simulink model "multirotor_simulation"  (R2025b)
settings: Solver=ode4  StartTime=0.0  StopTime=21  FixedStep=ST  RelTol=1e-3
values from neighbouring files (symbols this model uses):
  a0 = 0    [multirotor_start.m]
  ASLOPE = 5.9    [multirotor_start.m]
  Ax = 0.023    [multirotor_start.m]
  Ay = 0.023    [multirotor_start.m]
  Az = 0.106    [multirotor_start.m]
  BLADES = 2    [multirotor_start.m]
  BLCG = 0    [multirotor_start.m]
  BLCP = 0    [multirotor_start.m]
  BLH1 = b*sind(30)    [multirotor_start.m]
  BLH2 = b    (= 0.275)    [multirotor_start.m]
  BLH3 = b*sind(30)    [multirotor_start.m]
  BLH4 = -b*sind(30)    [multirotor_start.m]
  BLH5 = -b    (= -0.275)    [multirotor_start.m]
  BLH6 = -b*sind(30)    [multirotor_start.m]
  chi1 = 1    [multirotor_start.m]
  chi2 = -1    [multirotor_start.m]
  chi3 = 1    [multirotor_start.m]
  chi4 = -1    [multirotor_start.m]
  chi5 = 1    [multirotor_start.m]
  chi6 = -1    [multirotor_start.m]
  CHORD = 17.55e-3    (= 0.01755)    [multirotor_start.m]
  CHORD75 = 21e-3    (= 0.021)    [multirotor_start.m]
  controller_mode = 1    [multirotor_start.m]
  del_sp = [0 0.7 0 0]'    [multirotor_start.m]
  dyn_visco = 17.89e-6    (= 1.789e-05)    [multirotor_start.m]
  g0 = 9.80665    [multirotor_start.m]
  href = 0    [multirotor_start.m]
  k_ind = 1.35    [multirotor_start.m]
  k_Omega = 14.92    [multirotor_start.m]
  latref = 44.200626    [multirotor_start.m]
  lonref = 12.063822    [multirotor_start.m]
  m = 2.15    [multirotor_start.m]
  MC_ATT_PITCH = 30*pi/180    (= 0.523598775598)    [multirotor_start.m]
  MC_ATT_ROLL = 30*pi/180    (= 0.523598775598)    [multirotor_start.m]
  MC_ATT_YAW = 180*pi/180    (= 3.14159265359)    [multirotor_start.m]
  MC_PITCH_P = 3    [multirotor_start.m]
  MC_PITCHRATE_D = 0    [multirotor_start.m]
  MC_PITCHRATE_I = 0.1*0.5    (= 0.05)    [multirotor_start.m]
  MC_PITCHRATE_P = 0.09    [multirotor_start.m]
  MC_ROLL_P = 3    [multirotor_start.m]
  MC_ROLLRATE_D = 0    [multirotor_start.m]
  MC_ROLLRATE_I = 0.1*0.5    (= 0.05)    [multirotor_start.m]
  MC_ROLLRATE_P = 0.09    [multirotor_start.m]
  MC_VEL_FWD = 5    [multirotor_start.m]
  MC_VEL_FWD_OPT = 0.5    [multirotor_start.m]
  MC_VEL_LAT = 5    [multirotor_start.m]
  MC_VEL_LAT_OPT = 0.5    [multirotor_start.m]
  MC_VEL_VERT = 1    [multirotor_start.m]
  MC_YAW_P = 1.8*0.5    (= 0.9)    [multirotor_start.m]
  MC_YAWRATE_D = 0    [multirotor_start.m]
  MC_YAWRATE_I = 0.1*0    (= 0)    [multirotor_start.m]
  MC_YAWRATE_P = 0.175*0.4    (= 0.07)    [multirotor_start.m]
  MPC_XY_VEL_D_ACC = 0.2*2    (= 0.4)    [multirotor_start.m]
  MPC_XY_VEL_I_ACC = 0.8    [multirotor_start.m]
  MPC_XY_VEL_P_ACC = 1.7*3/3    (= 1.7)    [multirotor_start.m]
  MPC_Z_VEL_D_ACC = 0    [multirotor_start.m]
  MPC_Z_VEL_I_ACC = 2    [multirotor_start.m]
  MPC_Z_VEL_P_ACC = 4    [multirotor_start.m]
  n = 0.6359    [multirotor_start.m]
  p00 = 7.145e-2    (= 0.07145)    [multirotor_start.m]
  p01 = 0.4377    [multirotor_start.m]
  p02 = -10.13    [multirotor_start.m]
  p10 = 1.259e-3    (= 0.001259)    [multirotor_start.m]
  p11 = 1.284e-3    (= 0.001284)    [multirotor_start.m]
  p20 = -7.513e-7    (= -7.513e-07)    [multirotor_start.m]
  PWM_hover = (PWM_idle+PWM_max)/2    (= 1550)    [multirotor_start.m]
  PWM_idle = 1100    [multirotor_start.m]
  PWM_max = 2000    [multirotor_start.m]
  ROTOR = 4*0.0254    (= 0.1016)    [multirotor_start.m]
  set_point_input = 0    [multirotor_start.m]
  ST = 0.01    [multirotor_start.m]
  STACG = 0    [multirotor_start.m]
  STACP = 0    [multirotor_start.m]
  STAH1 = -b*cosd(30)    [multirotor_start.m]
  STAH2 = 0    [multirotor_start.m]
  STAH3 = b*cosd(30)    [multirotor_start.m]
  STAH4 = b*cosd(30)    [multirotor_start.m]
  STAH5 = 0    [multirotor_start.m]
  STAH6 = -b*cosd(30)    [multirotor_start.m]
  TERMINAL_SPEED = 0.5    [multirotor_start.m]
  Theta0 = 45*pi/180    (= 0.785398163397)    [multirotor_start.m]
  THETT = -38.0973*pi/180    (= -0.66492332112)    [multirotor_start.m]
  V_sin_x = 0.3    [multirotor_start.m]
  Vsp = [0 1 0]'    [multirotor_start.m]
  wind_rate = [0 0 0]'    [multirotor_start.m]
  wind_velocity_e = [0 0 0]'    [multirotor_start.m]
  WLCG = -0.03    [multirotor_start.m]
  WLCP = -0.08    [multirotor_start.m]
  WLH1 = 32e-3    (= 0.032)    [multirotor_start.m]
  WLH2 = 32e-3    (= 0.032)    [multirotor_start.m]
  WLH3 = 32e-3    (= 0.032)    [multirotor_start.m]
  WLH4 = 32e-3    (= 0.032)    [multirotor_start.m]
  WLH5 = 32e-3    (= 0.032)    [multirotor_start.m]
  WLH6 = 32e-3    (= 0.032)    [multirotor_start.m]
  Xe_target = Xe_0 + [2, 3, -10]'    [multirotor_start.m]
undefined symbols (not defined in the file or in its folder): fspecial, gray, Rec, SDTV, Sim3dSensor, X, Y, Z
libraries: sm_lib x258, slpidlib x18, nesl_utility x15, sharedtransform x4, simulink x3, aerolibanimutils x2, sim3dcameralib x2, dspvision x2, uavsim3dlib x2, aerolibutil x2, visionconversions x1, visionanalysis x1
(part 9 of 10)

== system multirotor_simulation/MULTIROTOR/3D/SIMECHANICS 3D SCENE/SimMechanics/MotorC/DCBL_Assembly_Clockwise_3_Top_1_RIGID/Assem3DCBL_Assembly_Clockwise_3_Top_1_RIGID ==
  Mieng_chan_canh_quat_1_RIGID : Subsystem
  ReferenceFrame : sm_lib/Frames and Transforms/Reference Frame
  Tang_tren_DCBL_1_RIGID : Subsystem
  Transform : sm_lib/Frames and Transforms/Rigid Transform  TranslationMethod=None  TranslationStandardOffset=0  TranslationStandardOffsetUnits=m  TranslationStandardAxis=+Z  TranslationCartesianOffset=[0 0 0]  TranslationCartesianOffsetUnits=m  TranslationROffset=0  TranslationROffsetUnits=m  TranslationZOffset=0  TranslationZOffsetUnits=m  TranslationThetaOffset=0  TranslationThetaOffsetUnits=deg  RotationMethod=None  RotationAngleUnits=deg  RotationStandardAxis=+Z  RotationAngle=0  RotationArbitraryAxis=[0 0 1]  FollAlignAxisA=+X  BaseAlignAxisA=+Y  FollAlignAxisB=+Y  BaseAlignAxisB=+Z  RotationSequenceAxes=FollowerAxes  RotationSequence=XYX  RotationSequenceAngles=[0 0 0]  RotationSequenceAnglesUnits=deg  RotationMatrix=[1 0 0; 0 1 0; 0 0 1]  Quaternion=[1 0 0 0]
  Transform1 : sm_lib/Frames and Transforms/Rigid Transform  TranslationMethod=Cartesian  TranslationStandardOffset=0  TranslationStandardOffsetUnits=mm  TranslationStandardAxis=+Z  TranslationCartesianOffset=[5.0000000000000044 5.5000000000000053 3.8000000000000256]  TranslationCartesianOffsetUnits=mm  TranslationROffset=0  TranslationROffsetUnits=m  TranslationZOffset=0  TranslationZOffsetUnits=m  TranslationThetaOffset=0  TranslationThetaOffsetUnits=deg  RotationMethod=ArbitraryAxis  RotationAngleUnits=rad  RotationStandardAxis=+Z  RotationAngle=3.1415926535897931  RotationArbitraryAxis=[0 1 0]  FollAlignAxisA=+X  BaseAlignAxisA=+Y  FollAlignAxisB=+Y  BaseAlignAxisB=+Z  RotationSequenceAxes=FollowerAxes  RotationSequence=XYX  RotationSequenceAngles=[0 0 0]  RotationSequenceAnglesUnits=deg  RotationMatrix=[1 0 0; 0 1 0; 0 0 1]  Quaternion=[1 0 0 0]
  Transform2 : sm_lib/Frames and Transforms/Rigid Transform  TranslationMethod=Cartesian  TranslationStandardOffset=0  TranslationStandardOffsetUnits=mm  TranslationStandardAxis=+Z  TranslationCartesianOffset=[0 12.200000000000017 0]  TranslationCartesianOffsetUnits=mm  TranslationROffset=0  TranslationROffsetUnits=m  TranslationZOffset=0  TranslationZOffsetUnits=m  TranslationThetaOffset=0  TranslationThetaOffsetUnits=deg  RotationMethod=ArbitraryAxis  RotationAngleUnits=rad  RotationStandardAxis=+Z  RotationAngle=3.1415926535897931  RotationArbitraryAxis=[0 1 0]  FollAlignAxisA=+X  BaseAlignAxisA=+Y  FollAlignAxisB=+Y  BaseAlignAxisB=+Z  RotationSequenceAxes=FollowerAxes  RotationSequence=XYX  RotationSequenceAngles=[0 0 0]  RotationSequenceAnglesUnits=deg  RotationMatrix=[1 0 0; 0 1 0; 0 0 1]  Quaternion=[1 0 0 0]
  Transform3 : sm_lib/Frames and Transforms/Rigid Transform  TranslationMethod=Cartesian  TranslationStandardOffset=0  TranslationStandardOffsetUnits=mm  TranslationStandardAxis=+Z  TranslationCartesianOffset=[0 16.899999999999999 0]  TranslationCartesianOffsetUnits=mm  TranslationROffset=0  TranslationROffsetUnits=m  TranslationZOffset=0  TranslationZOffsetUnits=m  TranslationThetaOffset=0  TranslationThetaOffsetUnits=deg  RotationMethod=ArbitraryAxis  RotationAngleUnits=rad  RotationStandardAxis=+Z  RotationAngle=2.0943951023931957  RotationArbitraryAxis=[-0.57735026918962562 0.57735026918962573 0.57735026918962573]  FollAlignAxisA=+X  BaseAlignAxisA=+Y  FollAlignAxisB=+Y  BaseAlignAxisB=+Z  RotationSequenceAxes=FollowerAxes  RotationSequence=XYX  RotationSequenceAngles=[0 0 0]  RotationSequenceAnglesUnits=deg  RotationMatrix=[1 0 0; 0 1 0; 0 0 1]  Quaternion=[1 0 0 0]
  Transform4 : sm_lib/Frames and Transforms/Rigid Transform  TranslationMethod=Cartesian  TranslationStandardOffset=0  TranslationStandardOffsetUnits=mm  TranslationStandardAxis=+Z  TranslationCartesianOffset=[0 30.500000000000014 0]  TranslationCartesianOffsetUnits=mm  TranslationROffset=0  TranslationROffsetUnits=m  TranslationZOffset=0  TranslationZOffsetUnits=m  TranslationThetaOffset=0  TranslationThetaOffsetUnits=deg  RotationMethod=ArbitraryAxis  RotationAngleUnits=rad  RotationStandardAxis=+Z  RotationAngle=2.994911156014171  RotationArbitraryAxis=[0 1 0]  FollAlignAxisA=+X  BaseAlignAxisA=+Y  FollAlignAxisB=+Y  BaseAlignAxisB=+Z  RotationSequenceAxes=FollowerAxes  RotationSequence=XYX  RotationSequenceAngles=[0 0 0]  RotationSequenceAnglesUnits=deg  RotationMatrix=[1 0 0; 0 1 0; 0 0 1]  Quaternion=[1 0 0 0]
  hex_nut_style_1_gradeab_iso_1_RIGID : Subsystem
  x10x4_7_clockwise_propeller_1_RIGID : Subsystem
  F : PMIOPort  Side=Left
  connections:
  Tang_tren_DCBL_1_RIGID/LConn1 -- Transform/RConn1
  Transform1/RConn1 -- x10x4_7_clockwise_propeller_1_RIGID/LConn1
  Mieng_chan_canh_quat_1_RIGID/LConn1 -- Transform2/RConn1
  Transform3/RConn1 -- hex_nut_style_1_gradeab_iso_1_RIGID/LConn1
  Transform/LConn1 -- ReferenceFrame/RConn1 -- Transform1/LConn1 -- Transform2/LConn1 -- Transform3/LConn1 -- Transform4/RConn1
  Transform4/LConn1 -- F/RConn1

== system multirotor_simulation/MULTIROTOR/3D/SIMECHANICS 3D SCENE/SimMechanics/MotorD/DCBL_Assembly_CounterClockwise_4_Top_1_RIGID/Assem4DCBL_Assembly_CounterClockwise_4_Top_1_RIGID ==
  Mieng_chan_canh_quat_1_RIGID : Subsystem
  ReferenceFrame : sm_lib/Frames and Transforms/Reference Frame
  Tang_tren_DCBL_1_RIGID : Subsystem
  Transform : sm_lib/Frames and Transforms/Rigid Transform  TranslationMethod=None  TranslationStandardOffset=0  TranslationStandardOffsetUnits=m  TranslationStandardAxis=+Z  TranslationCartesianOffset=[0 0 0]  TranslationCartesianOffsetUnits=m  TranslationROffset=0  TranslationROffsetUnits=m  TranslationZOffset=0  TranslationZOffsetUnits=m  TranslationThetaOffset=0  TranslationThetaOffsetUnits=deg  RotationMethod=None  RotationAngleUnits=deg  RotationStandardAxis=+Z  RotationAngle=0  RotationArbitraryAxis=[0 0 1]  FollAlignAxisA=+X  BaseAlignAxisA=+Y  FollAlignAxisB=+Y  BaseAlignAxisB=+Z  RotationSequenceAxes=FollowerAxes  RotationSequence=XYX  RotationSequenceAngles=[0 0 0]  RotationSequenceAnglesUnits=deg  RotationMatrix=[1 0 0; 0 1 0; 0 0 1]  Quaternion=[1 0 0 0]
  Transform1 : sm_lib/Frames and Transforms/Rigid Transform  TranslationMethod=Cartesian  TranslationStandardOffset=0  TranslationStandardOffsetUnits=mm  TranslationStandardAxis=+Z  TranslationCartesianOffset=[0 12.200000000000017 0]  TranslationCartesianOffsetUnits=mm  TranslationROffset=0  TranslationROffsetUnits=m  TranslationZOffset=0  TranslationZOffsetUnits=m  TranslationThetaOffset=0  TranslationThetaOffsetUnits=deg  RotationMethod=ArbitraryAxis  RotationAngleUnits=rad  RotationStandardAxis=+Z  RotationAngle=3.1415926535897931  RotationArbitraryAxis=[0 1 0]  FollAlignAxisA=+X  BaseAlignAxisA=+Y  FollAlignAxisB=+Y  BaseAlignAxisB=+Z  RotationSequenceAxes=FollowerAxes  RotationSequence=XYX  RotationSequenceAngles=[0 0 0]  RotationSequenceAnglesUnits=deg  RotationMatrix=[1 0 0; 0 1 0; 0 0 1]  Quaternion=[1 0 0 0]
  Transform2 : sm_lib/Frames and Transforms/Rigid Transform  TranslationMethod=Cartesian  TranslationStandardOffset=0  TranslationStandardOffsetUnits=mm  TranslationStandardAxis=+Z  TranslationCartesianOffset=[5.0000000000000044 5.5000000000000053 3.8000000000000118]  TranslationCartesianOffsetUnits=mm  TranslationROffset=0  TranslationROffsetUnits=m  TranslationZOffset=0  TranslationZOffsetUnits=m  TranslationThetaOffset=0  TranslationThetaOffsetUnits=deg  RotationMethod=ArbitraryAxis  RotationAngleUnits=rad  RotationStandardAxis=+Z  RotationAngle=3.1415926535897931  RotationArbitraryAxis=[0 1 0]  FollAlignAxisA=+X  BaseAlignAxisA=+Y  FollAlignAxisB=+Y  BaseAlignAxisB=+Z  RotationSequenceAxes=FollowerAxes  RotationSequence=XYX  RotationSequenceAngles=[0 0 0]  RotationSequenceAnglesUnits=deg  RotationMatrix=[1 0 0; 0 1 0; 0 0 1]  Quaternion=[1 0 0 0]
  Transform3 : sm_lib/Frames and Transforms/Rigid Transform  TranslationMethod=Cartesian  TranslationStandardOffset=0  TranslationStandardOffsetUnits=mm  TranslationStandardAxis=+Z  TranslationCartesianOffset=[0 16.899999999999999 0]  TranslationCartesianOffsetUnits=mm  TranslationROffset=0  TranslationROffsetUnits=m  TranslationZOffset=0  TranslationZOffsetUnits=m  TranslationThetaOffset=0  TranslationThetaOffsetUnits=deg  RotationMethod=ArbitraryAxis  RotationAngleUnits=rad  RotationStandardAxis=+Z  RotationAngle=2.0943951023931953  RotationArbitraryAxis=[-0.57735026918962584 0.57735026918962584 0.57735026918962584]  FollAlignAxisA=+X  BaseAlignAxisA=+Y  FollAlignAxisB=+Y  BaseAlignAxisB=+Z  RotationSequenceAxes=FollowerAxes  RotationSequence=XYX  RotationSequenceAngles=[0 0 0]  RotationSequenceAnglesUnits=deg  RotationMatrix=[1 0 0; 0 1 0; 0 0 1]  Quaternion=[1 0 0 0]
  Transform4 : sm_lib/Frames and Transforms/Rigid Transform  TranslationMethod=Cartesian  TranslationStandardOffset=0  TranslationStandardOffsetUnits=mm  TranslationStandardAxis=+Z  TranslationCartesianOffset=[0 30.500000000000014 0]  TranslationCartesianOffsetUnits=mm  TranslationROffset=0  TranslationROffsetUnits=m  TranslationZOffset=0  TranslationZOffsetUnits=m  TranslationThetaOffset=0  TranslationThetaOffsetUnits=deg  RotationMethod=ArbitraryAxis  RotationAngleUnits=rad  RotationStandardAxis=+Z  RotationAngle=2.994911156014171  RotationArbitraryAxis=[0 1 0]  FollAlignAxisA=+X  BaseAlignAxisA=+Y  FollAlignAxisB=+Y  BaseAlignAxisB=+Z  RotationSequenceAxes=FollowerAxes  RotationSequence=XYX  RotationSequenceAngles=[0 0 0]  RotationSequenceAnglesUnits=deg  RotationMatrix=[1 0 0; 0 1 0; 0 0 1]  Quaternion=[1 0 0 0]
  hex_nut_style_1_gradeab_iso_1_RIGID : Subsystem
  x10x4_7_counterclockwise_propeller_1_RIGID : Subsystem
  F : PMIOPort  Side=Left
  connections:
  Tang_tren_DCBL_1_RIGID/LConn1 -- Transform/RConn1
  Mieng_chan_canh_quat_1_RIGID/LConn1 -- Transform1/RConn1
  Transform2/RConn1 -- x10x4_7_counterclockwise_propeller_1_RIGID/LConn1
  Transform3/RConn1 -- hex_nut_style_1_gradeab_iso_1_RIGID/LConn1
  Transform/LConn1 -- Transform1/LConn1 -- Transform4/RConn1 -- ReferenceFrame/RConn1 -- Transform2/LConn1 -- Transform3/LConn1
  Transform4/LConn1 -- F/RConn1

== system multirotor_simulation/MULTIROTOR/3D/SIMECHANICS 3D SCENE/SimMechanics/Assembly_Quadrotor_NProp_1_RIGID/Assembly_Quadrotor_NoProp_1_RIGID/DCBL_Assembly_Clockwise_1_Bottom_1_RIGID/De_DCBL_1_RIGID ==
  ReferenceFrame : sm_lib/Frames and Transforms/Reference Frame
  Solid : sm_lib/Body Elements/File Solid  ExtGeomFileName=De_DCBL_Default_sldprt.STL  UnitType=Custom  ExtGeomFileUnits=mm  StepReaderType=HEX  ExportConvexHullGeometry=off  InertiaType=Custom  Mass=0.0094405067370886605  MassUnits=kg  CenterOfMass=[0 8.551755407943574 0]  CenterOfMassUnits=mm  MomentsOfInertia=[0.9581719720589793 0.57744869492610285 0.95817197205897908]  MomentsOfInertiaUnits=kg*mm^2  ProductsOfInertia=[0 -0.0012524646336928653 0]  ProductsOfInertiaUnits=kg*mm^2  BasedOnType=Density  Density=1000  DensityUnits=kg/(m^3)  DoExposeReferenceFrame=on  SerializedFrames=<Frames/>  GraphicType=FromGeometry  MarkerShape=Sphere  MarkerSize=10  MarkerSizeUnits=m  GraphicVisPropType=SimpleVisualProperties  GraphicDiffuseColor=[0.2 0.2 0.2]  GraphicSpecularColor=[0.5 0.5 0.5 1.0]  GraphicAmbientColor=[0.15 0.15 0.15 1.0]  GraphicEmissiveColor=[0.0 0.0 0.0 1.0]  GraphicShininess=75  GraphicOpacity=1
  F : PMIOPort  Side=Left
  connections:
  Solid/RConn1 -- ReferenceFrame/RConn1 -- F/RConn1

== system multirotor_simulation/MULTIROTOR/3D/SIMECHANICS 3D SCENE/SimMechanics/Assembly_Quadrotor_NProp_1_RIGID/Assembly_Quadrotor_NoProp_1_RIGID/DCBL_Assembly_Clockwise_3_Bottom_1_RIGID/De_DCBL_1_RIGID ==
  ReferenceFrame : sm_lib/Frames and Transforms/Reference Frame
  Solid : sm_lib/Body Elements/File Solid  ExtGeomFileName=De_DCBL_Default_sldprt.STL  UnitType=Custom  ExtGeomFileUnits=mm  StepReaderType=HEX  ExportConvexHullGeometry=off  InertiaType=Custom  Mass=0.0094405067370886605  MassUnits=kg  CenterOfMass=[0 8.551755407943574 0]  CenterOfMassUnits=mm  MomentsOfInertia=[0.9581719720589793 0.57744869492610285 0.95817197205897908]  MomentsOfInertiaUnits=kg*mm^2  ProductsOfInertia=[0 -0.0012524646336928653 0]  ProductsOfInertiaUnits=kg*mm^2  BasedOnType=Density  Density=1000  DensityUnits=kg/(m^3)  DoExposeReferenceFrame=on  SerializedFrames=<Frames/>  GraphicType=FromGeometry  MarkerShape=Sphere  MarkerSize=10  MarkerSizeUnits=m  GraphicVisPropType=SimpleVisualProperties  GraphicDiffuseColor=[0.2 0.2 0.2]  GraphicSpecularColor=[0.5 0.5 0.5 1.0]  GraphicAmbientColor=[0.15 0.15 0.15 1.0]  GraphicEmissiveColor=[0.0 0.0 0.0 1.0]  GraphicShininess=75  GraphicOpacity=1
  F : PMIOPort  Side=Left
  connections:
  Solid/RConn1 -- ReferenceFrame/RConn1 -- F/RConn1

== system multirotor_simulation/MULTIROTOR/3D/SIMECHANICS 3D SCENE/SimMechanics/Assembly_Quadrotor_NProp_1_RIGID/Assembly_Quadrotor_NoProp_1_RIGID/DCBL_Assembly_CounterClockwise_2_Bottom_1_RIGID/De_DCBL_1_RIGID ==
  ReferenceFrame : sm_lib/Frames and Transforms/Reference Frame
  Solid : sm_lib/Body Elements/File Solid  ExtGeomFileName=De_DCBL_Default_sldprt.STL  UnitType=Custom  ExtGeomFileUnits=mm  StepReaderType=HEX  ExportConvexHullGeometry=off  InertiaType=Custom  Mass=0.0094405067370886605  MassUnits=kg  CenterOfMass=[0 8.551755407943574 0]  CenterOfMassUnits=mm  MomentsOfInertia=[0.9581719720589793 0.57744869492610285 0.95817197205897908]  MomentsOfInertiaUnits=kg*mm^2  ProductsOfInertia=[0 -0.0012524646336928653 0]  ProductsOfInertiaUnits=kg*mm^2  BasedOnType=Density  Density=1000  DensityUnits=kg/(m^3)  DoExposeReferenceFrame=on  SerializedFrames=<Frames/>  GraphicType=FromGeometry  MarkerShape=Sphere  MarkerSize=10  MarkerSizeUnits=m  GraphicVisPropType=SimpleVisualProperties  GraphicDiffuseColor=[0.2 0.2 0.2]  GraphicSpecularColor=[0.5 0.5 0.5 1.0]  GraphicAmbientColor=[0.15 0.15 0.15 1.0]  GraphicEmissiveColor=[0.0 0.0 0.0 1.0]  GraphicShininess=75  GraphicOpacity=1
  F : PMIOPort  Side=Left
  connections:
  Solid/RConn1 -- ReferenceFrame/RConn1 -- F/RConn1

== system multirotor_simulation/MULTIROTOR/3D/SIMECHANICS 3D SCENE/SimMechanics/Assembly_Quadrotor_NProp_1_RIGID/Assembly_Quadrotor_NoProp_1_RIGID/DCBL_Assembly_CounterClockwise_4_Bottom_1_RIGID/De_DCBL_1_RIGID ==
  ReferenceFrame : sm_lib/Frames and Transforms/Reference Frame
  Solid : sm_lib/Body Elements/File Solid  ExtGeomFileName=De_DCBL_Default_sldprt.STL  UnitType=Custom  ExtGeomFileUnits=mm  StepReaderType=HEX  ExportConvexHullGeometry=off  InertiaType=Custom  Mass=0.0094405067370886605  MassUnits=kg  CenterOfMass=[0 8.551755407943574 0]  CenterOfMassUnits=mm  MomentsOfInertia=[0.9581719720589793 0.57744869492610285 0.95817197205897908]  MomentsOfInertiaUnits=kg*mm^2  ProductsOfInertia=[0 -0.0012524646336928653 0]  ProductsOfInertiaUnits=kg*mm^2  BasedOnType=Density  Density=1000  DensityUnits=kg/(m^3)  DoExposeReferenceFrame=on  SerializedFrames=<Frames/>  GraphicType=FromGeometry  MarkerShape=Sphere  MarkerSize=10  MarkerSizeUnits=m  GraphicVisPropType=SimpleVisualProperties  GraphicDiffuseColor=[0.2 0.2 0.2]  GraphicSpecularColor=[0.5 0.5 0.5 1.0]  GraphicAmbientColor=[0.15 0.15 0.15 1.0]  GraphicEmissiveColor=[0.0 0.0 0.0 1.0]  GraphicShininess=75  GraphicOpacity=1
  F : PMIOPort  Side=Left
  connections:
  Solid/RConn1 -- ReferenceFrame/RConn1 -- F/RConn1

== system multirotor_simulation/MULTIROTOR/3D/SIMECHANICS 3D SCENE/SimMechanics/MotorA/DCBL_Assembly_Clockwise_1_Top_1_RIGID/Assem1DCBL_Assembly_Clockwise_1_Top_1_RIGID/Mieng_chan_canh_quat_1_RIGID ==
  ReferenceFrame : sm_lib/Frames and Transforms/Reference Frame
  Solid : sm_lib/Body Elements/File Solid  ExtGeomFileName=Mieng_chan_canh_quat_Default_sldprt.STL  UnitType=Custom  ExtGeomFileUnits=mm  StepReaderType=HEX  ExportConvexHullGeometry=off  InertiaType=Custom  Mass=0.00066710164886432991  MassUnits=kg  CenterOfMass=[0 0.34100350204192958 0]  CenterOfMassUnits=mm  MomentsOfInertia=[0.0086037825507957657 0.016809111968954363 0.0086037825507957692]  MomentsOfInertiaUnits=kg*mm^2  ProductsOfInertia=[0 0 0]  ProductsOfInertiaUnits=kg*mm^2  BasedOnType=Density  Density=1000  DensityUnits=kg/(m^3)  DoExposeReferenceFrame=on  SerializedFrames=<Frames/>  GraphicType=FromGeometry  MarkerShape=Sphere  MarkerSize=10  MarkerSizeUnits=m  GraphicVisPropType=SimpleVisualProperties  GraphicDiffuseColor=[0.1 0.1 0.1]  GraphicSpecularColor=[0.5 0.5 0.5 1.0]  GraphicAmbientColor=[0.15 0.15 0.15 1.0]  GraphicEmissiveColor=[0.0 0.0 0.0 1.0]  GraphicShininess=75  GraphicOpacity=1
  F : PMIOPort  Side=Left
  connections:
  Solid/RConn1 -- ReferenceFrame/RConn1 -- F/RConn1

== system multirotor_simulation/MULTIROTOR/3D/SIMECHANICS 3D SCENE/SimMechanics/MotorA/DCBL_Assembly_Clockwise_1_Top_1_RIGID/Assem1DCBL_Assembly_Clockwise_1_Top_1_RIGID/Tang_tren_DCBL_1_RIGID ==
  ReferenceFrame : sm_lib/Frames and Transforms/Reference Frame
  Solid : sm_lib/Body Elements/File Solid  ExtGeomFileName=Tang_tren_DCBL_Default_sldprt.STL  UnitType=Custom  ExtGeomFileUnits=mm  StepReaderType=HEX  ExportConvexHullGeometry=off  InertiaType=Custom  Mass=0.0096533797201190392  MassUnits=kg  CenterOfMass=[0 -3.2502099324489322 0]  CenterOfMassUnits=mm  MomentsOfInertia=[1.2743807926810715 0.81038583319969226 1.2743807926810709]  MomentsOfInertiaUnits=kg*mm^2  ProductsOfInertia=[0 0 0]  ProductsOfInertiaUnits=kg*mm^2  BasedOnType=Density  Density=1000  DensityUnits=kg/(m^3)  DoExposeReferenceFrame=on  SerializedFrames=<Frames/>  GraphicType=FromGeometry  MarkerShape=Sphere  MarkerSize=10  MarkerSizeUnits=m  GraphicVisPropType=SimpleVisualProperties  GraphicDiffuseColor=[0.1 0.1 0.1]  GraphicSpecularColor=[0.5 0.5 0.5 1.0]  GraphicAmbientColor=[0.15 0.15 0.15 1.0]  GraphicEmissiveColor=[0.0 0.0 0.0 1.0]  GraphicShininess=75  GraphicOpacity=1
  F : PMIOPort  Side=Left
  connections:
  Solid/RConn1 -- ReferenceFrame/RConn1 -- F/RConn1

== system multirotor_simulation/MULTIROTOR/3D/SIMECHANICS 3D SCENE/SimMechanics/MotorA/DCBL_Assembly_Clockwise_1_Top_1_RIGID/Assem1DCBL_Assembly_Clockwise_1_Top_1_RIGID/hex_nut_style_1_gradeab_iso_1_RIGID ==
  ReferenceFrame : sm_lib/Frames and Transforms/Reference Frame
  Solid : sm_lib/Body Elements/File Solid  ExtGeomFileName=hex nut style 1 gradeab_iso_Hexagon Nut ISO - 4032 - M4 - D - N_sldprt.STL  UnitType=Custom  ExtGeomFileUnits=mm  StepReaderType=HEX  ExportConvexHullGeometry=off  InertiaType=Custom  Mass=0.00010662444846940384  MassUnits=kg  CenterOfMass=[0 1.3702747535691162e-06 -1.5985959803450969]  CenterOfMassUnits=mm  MomentsOfInertia=[0.00052487586358693401 0.00052487294180577238 0.00087302244809774987]  MomentsOfInertiaUnits=kg*mm^2  ProductsOfInertia=[0 0 0]  ProductsOfInertiaUnits=kg*mm^2  BasedOnType=Density  Density=1000  DensityUnits=kg/(m^3)  DoExposeReferenceFrame=on  SerializedFrames=<Frames/>  GraphicType=FromGeometry  MarkerShape=Sphere  MarkerSize=10  MarkerSizeUnits=m  GraphicVisPropType=SimpleVisualProperties  GraphicDiffuseColor=[0.77647058823529413 0.75686274509803919 0.73725490196078436]  GraphicSpecularColor=[0.5 0.5 0.5 1.0]  GraphicAmbientColor=[0.15 0.15 0.15 1.0]  GraphicEmissiveColor=[0.0 0.0 0.0 1.0]  GraphicShininess=75  GraphicOpacity=1
  F : PMIOPort  Side=Left
  connections:
  Solid/RConn1 -- ReferenceFrame/RConn1 -- F/RConn1

== system multirotor_simulation/MULTIROTOR/3D/SIMECHANICS 3D SCENE/SimMechanics/MotorA/DCBL_Assembly_Clockwise_1_Top_1_RIGID/Assem1DCBL_Assembly_Clockwise_1_Top_1_RIGID/x10x4_7_clockwise_propeller_1_RIGID ==
  ReferenceFrame : sm_lib/Frames and Transforms/Reference Frame
  Solid : sm_lib/Body Elements/File Solid  ExtGeomFileName=10x4.7-clockwise-propeller_Default_sldprt.STL  UnitType=Custom  ExtGeomFileUnits=mm  StepReaderType=HEX  ExportConvexHullGeometry=off  InertiaType=Custom  Mass=0.0085886554018527825  MassUnits=kg  CenterOfMass=[5.0000101361481475 5.1432840109255382 3.799999228152465]  CenterOfMassUnits=mm  MomentsOfInertia=[37.986675876119939 39.040615812058284 1.1185316341050053]  MomentsOfInertiaUnits=kg*mm^2  ProductsOfInertia=[-7.8946012766185134e-07 -5.513228057178063 2.3221541821947674e-07]  ProductsOfInertiaUnits=kg*mm^2  BasedOnType=Density  Density=1000  DensityUnits=kg/(m^3)  DoExposeReferenceFrame=on  SerializedFrames=<Frames/>  GraphicType=FromGeometry  MarkerShape=Sphere  MarkerSize=10  MarkerSizeUnits=m  GraphicVisPropType=SimpleVisualProperties  GraphicDiffuseColor=[0.75294117647058822 0.75294117647058822 0.75294117647058822]  GraphicSpecularColor=[0.5 0.5 0.5 1.0]  GraphicAmbientColor=[0.15 0.15 0.15 1.0]  GraphicEmissiveColor=[0.0 0.0 0.0 1.0]  GraphicShininess=75  GraphicOpacity=1
  F : PMIOPort  Side=Left
  connections:
  Solid/RConn1 -- ReferenceFrame/RConn1 -- F/RConn1

== system multirotor_simulation/MULTIROTOR/3D/SIMECHANICS 3D SCENE/SimMechanics/MotorB/DCBL_Assembly_CounterClockwise_2_Top_1_RIGID/Assem2DCBL_Assembly_CounterClockwise_2_Top_1_RIGID/Mieng_chan_canh_quat_1_RIGID ==
  ReferenceFrame : sm_lib/Frames and Transforms/Reference Frame
  Solid : sm_lib/Body Elements/File Solid  ExtGeomFileName=Mieng_chan_canh_quat_Default_sldprt.STL  UnitType=Custom  ExtGeomFileUnits=mm  StepReaderType=HEX  ExportConvexHullGeometry=off  InertiaType=Custom  Mass=0.00066710164886432991  MassUnits=kg  CenterOfMass=[0 0.34100350204192958 0]  CenterOfMassUnits=mm  MomentsOfInertia=[0.0086037825507957657 0.016809111968954363 0.0086037825507957692]  MomentsOfInertiaUnits=kg*mm^2  ProductsOfInertia=[0 0 0]  ProductsOfInertiaUnits=kg*mm^2  BasedOnType=Density  Density=1000  DensityUnits=kg/(m^3)  DoExposeReferenceFrame=on  SerializedFrames=<Frames/>  GraphicType=FromGeometry  MarkerShape=Sphere  MarkerSize=10  MarkerSizeUnits=m  GraphicVisPropType=SimpleVisualProperties  GraphicDiffuseColor=[0.1 0.1 0.1]  GraphicSpecularColor=[0.5 0.5 0.5 1.0]  GraphicAmbientColor=[0.15 0.15 0.15 1.0]  GraphicEmissiveColor=[0.0 0.0 0.0 1.0]  GraphicShininess=75  GraphicOpacity=1
  F : PMIOPort  Side=Left
  connections:
  Solid/RConn1 -- ReferenceFrame/RConn1 -- F/RConn1

== system multirotor_simulation/MULTIROTOR/3D/SIMECHANICS 3D SCENE/SimMechanics/MotorB/DCBL_Assembly_CounterClockwise_2_Top_1_RIGID/Assem2DCBL_Assembly_CounterClockwise_2_Top_1_RIGID/Tang_tren_DCBL_1_RIGID ==
  ReferenceFrame : sm_lib/Frames and Transforms/Reference Frame
  Solid : sm_lib/Body Elements/File Solid  ExtGeomFileName=Tang_tren_DCBL_Default_sldprt.STL  UnitType=Custom  ExtGeomFileUnits=mm  StepReaderType=HEX  ExportConvexHullGeometry=off  InertiaType=Custom  Mass=0.0096533797201190392  MassUnits=kg  CenterOfMass=[0 -3.2502099324489322 0]  CenterOfMassUnits=mm  MomentsOfInertia=[1.2743807926810715 0.81038583319969226 1.2743807926810709]  MomentsOfInertiaUnits=kg*mm^2  ProductsOfInertia=[0 0 0]  ProductsOfInertiaUnits=kg*mm^2  BasedOnType=Density  Density=1000  DensityUnits=kg/(m^3)  DoExposeReferenceFrame=on  SerializedFrames=<Frames/>  GraphicType=FromGeometry  MarkerShape=Sphere  MarkerSize=10  MarkerSizeUnits=m  GraphicVisPropType=SimpleVisualProperties  GraphicDiffuseColor=[0.1 0.1 0.1]  GraphicSpecularColor=[0.5 0.5 0.5 1.0]  GraphicAmbientColor=[0.15 0.15 0.15 1.0]  GraphicEmissiveColor=[0.0 0.0 0.0 1.0]  GraphicShininess=75  GraphicOpacity=1
  F : PMIOPort  Side=Left
  connections:
  Solid/RConn1 -- ReferenceFrame/RConn1 -- F/RConn1

== system multirotor_simulation/MULTIROTOR/3D/SIMECHANICS 3D SCENE/SimMechanics/MotorB/DCBL_Assembly_CounterClockwise_2_Top_1_RIGID/Assem2DCBL_Assembly_CounterClockwise_2_Top_1_RIGID/hex_nut_style_1_gradeab_iso_1_RIGID ==
  ReferenceFrame : sm_lib/Frames and Transforms/Reference Frame
  Solid : sm_lib/Body Elements/File Solid  ExtGeomFileName=hex nut style 1 gradeab_iso_Hexagon Nut ISO - 4032 - M4 - D - N_sldprt.STL  UnitType=Custom  ExtGeomFileUnits=mm  StepReaderType=HEX  ExportConvexHullGeometry=off  InertiaType=Custom  Mass=0.00010662444846940384  MassUnits=kg  CenterOfMass=[0 1.3702747535691162e-06 -1.5985959803450969]  CenterOfMassUnits=mm  MomentsOfInertia=[0.00052487586358693401 0.00052487294180577238 0.00087302244809774987]  MomentsOfInertiaUnits=kg*mm^2  ProductsOfInertia=[0 0 0]  ProductsOfInertiaUnits=kg*mm^2  BasedOnType=Density  Density=1000  DensityUnits=kg/(m^3)  DoExposeReferenceFrame=on  SerializedFrames=<Frames/>  GraphicType=FromGeometry  MarkerShape=Sphere  MarkerSize=10  MarkerSizeUnits=m  GraphicVisPropType=SimpleVisualProperties  GraphicDiffuseColor=[0.77647058823529413 0.75686274509803919 0.73725490196078436]  GraphicSpecularColor=[0.5 0.5 0.5 1.0]  GraphicAmbientColor=[0.15 0.15 0.15 1.0]  GraphicEmissiveColor=[0.0 0.0 0.0 1.0]  GraphicShininess=75  GraphicOpacity=1
  F : PMIOPort  Side=Left
  connections:
  Solid/RConn1 -- ReferenceFrame/RConn1 -- F/RConn1

== system multirotor_simulation/MULTIROTOR/3D/SIMECHANICS 3D SCENE/SimMechanics/MotorB/DCBL_Assembly_CounterClockwise_2_Top_1_RIGID/Assem2DCBL_Assembly_CounterClockwise_2_Top_1_RIGID/x10x4_7_counterclockwise_propeller_1_RIGID ==
  ReferenceFrame : sm_lib/Frames and Transforms/Reference Frame
  Solid : sm_lib/Body Elements/File Solid  ExtGeomFileName=10x4.7-counterclockwise-propeller_Default_sldprt.STL  UnitType=Custom  ExtGeomFileUnits=mm  StepReaderType=HEX  ExportConvexHullGeometry=off  InertiaType=Custom  Mass=0.0086221636611543556  MassUnits=kg  CenterOfMass=[5.0000063702530122 5.136767030722547 3.7999863031218535]  CenterOfMassUnits=mm  MomentsOfInertia=[38.086408780943664 39.145966882895458 1.124519086575168]  MomentsOfInertiaUnits=kg*mm^2  ProductsOfInertia=[-1.7703894482553841e-07 5.5344154529569156 1.457353668708178e-07]  ProductsOfInertiaUnits=kg*mm^2  BasedOnType=Density  Density=1000  DensityUnits=kg/(m^3)  DoExposeReferenceFrame=on  SerializedFrames=<Frames/>  GraphicType=FromGeometry  MarkerShape=Sphere  MarkerSize=10  MarkerSizeUnits=m  GraphicVisPropType=SimpleVisualProperties  GraphicDiffuseColor=[0.75294117647058822 0.75294117647058822 0.75294117647058822]  GraphicSpecularColor=[0.5 0.5 0.5 1.0]  GraphicAmbientColor=[0.15 0.15 0.15 1.0]  GraphicEmissiveColor=[0.0 0.0 0.0 1.0]  GraphicShininess=75  GraphicOpacity=1
  F : PMIOPort  Side=Left
  connections:
  Solid/RConn1 -- ReferenceFrame/RConn1 -- F/RConn1

== system multirotor_simulation/MULTIROTOR/3D/SIMECHANICS 3D SCENE/SimMechanics/MotorC/DCBL_Assembly_Clockwise_3_Top_1_RIGID/Assem3DCBL_Assembly_Clockwise_3_Top_1_RIGID/Mieng_chan_canh_quat_1_RIGID ==
  ReferenceFrame : sm_lib/Frames and Transforms/Reference Frame
  Solid : sm_lib/Body Elements/File Solid  ExtGeomFileName=Mieng_chan_canh_quat_Default_sldprt.STL  UnitType=Custom  ExtGeomFileUnits=mm  StepReaderType=HEX  ExportConvexHullGeometry=off  InertiaType=Custom  Mass=0.00066710164886432991  MassUnits=kg  CenterOfMass=[0 0.34100350204192958 0]  CenterOfMassUnits=mm  MomentsOfInertia=[0.0086037825507957657 0.016809111968954363 0.0086037825507957692]  MomentsOfInertiaUnits=kg*mm^2  ProductsOfInertia=[0 0 0]  ProductsOfInertiaUnits=kg*mm^2  BasedOnType=Density  Density=1000  DensityUnits=kg/(m^3)  DoExposeReferenceFrame=on  SerializedFrames=<Frames/>  GraphicType=FromGeometry  MarkerShape=Sphere  MarkerSize=10  MarkerSizeUnits=m  GraphicVisPropType=SimpleVisualProperties  GraphicDiffuseColor=[0.1 0.1 0.1]  GraphicSpecularColor=[0.5 0.5 0.5 1.0]  GraphicAmbientColor=[0.15 0.15 0.15 1.0]  GraphicEmissiveColor=[0.0 0.0 0.0 1.0]  GraphicShininess=75  GraphicOpacity=1
  F : PMIOPort  Side=Left
  connections:
  Solid/RConn1 -- ReferenceFrame/RConn1 -- F/RConn1

== system multirotor_simulation/MULTIROTOR/3D/SIMECHANICS 3D SCENE/SimMechanics/MotorC/DCBL_Assembly_Clockwise_3_Top_1_RIGID/Assem3DCBL_Assembly_Clockwise_3_Top_1_RIGID/Tang_tren_DCBL_1_RIGID ==
  ReferenceFrame : sm_lib/Frames and Transforms/Reference Frame
  Solid : sm_lib/Body Elements/File Solid  ExtGeomFileName=Tang_tren_DCBL_Default_sldprt.STL  UnitType=Custom  ExtGeomFileUnits=mm  StepReaderType=HEX  ExportConvexHullGeometry=off  InertiaType=Custom  Mass=0.0096533797201190392  MassUnits=kg  CenterOfMass=[0 -3.2502099324489322 0]  CenterOfMassUnits=mm  MomentsOfInertia=[1.2743807926810715 0.81038583319969226 1.2743807926810709]  MomentsOfInertiaUnits=kg*mm^2  ProductsOfInertia=[0 0 0]  ProductsOfInertiaUnits=kg*mm^2  BasedOnType=Density  Density=1000  DensityUnits=kg/(m^3)  DoExposeReferenceFrame=on  SerializedFrames=<Frames/>  GraphicType=FromGeometry  MarkerShape=Sphere  MarkerSize=10  MarkerSizeUnits=m  GraphicVisPropType=SimpleVisualProperties  GraphicDiffuseColor=[0.1 0.1 0.1]  GraphicSpecularColor=[0.5 0.5 0.5 1.0]  GraphicAmbientColor=[0.15 0.15 0.15 1.0]  GraphicEmissiveColor=[0.0 0.0 0.0 1.0]  GraphicShininess=75  GraphicOpacity=1
  F : PMIOPort  Side=Left
  connections:
  Solid/RConn1 -- ReferenceFrame/RConn1 -- F/RConn1

== system multirotor_simulation/MULTIROTOR/3D/SIMECHANICS 3D SCENE/SimMechanics/MotorC/DCBL_Assembly_Clockwise_3_Top_1_RIGID/Assem3DCBL_Assembly_Clockwise_3_Top_1_RIGID/hex_nut_style_1_gradeab_iso_1_RIGID ==
  ReferenceFrame : sm_lib/Frames and Transforms/Reference Frame
  Solid : sm_lib/Body Elements/File Solid  ExtGeomFileName=hex nut style 1 gradeab_iso_Hexagon Nut ISO - 4032 - M4 - D - N_sldprt.STL  UnitType=Custom  ExtGeomFileUnits=mm  StepReaderType=HEX  ExportConvexHullGeometry=off  InertiaType=Custom  Mass=0.00010662444846940384  MassUnits=kg  CenterOfMass=[0 1.3702747535691162e-06 -1.5985959803450969]  CenterOfMassUnits=mm  MomentsOfInertia=[0.00052487586358693401 0.00052487294180577238 0.00087302244809774987]  MomentsOfInertiaUnits=kg*mm^2  ProductsOfInertia=[0 0 0]  ProductsOfInertiaUnits=kg*mm^2  BasedOnType=Density  Density=1000  DensityUnits=kg/(m^3)  DoExposeReferenceFrame=on  SerializedFrames=<Frames/>  GraphicType=FromGeometry  MarkerShape=Sphere  MarkerSize=10  MarkerSizeUnits=m  GraphicVisPropType=SimpleVisualProperties  GraphicDiffuseColor=[0.77647058823529413 0.75686274509803919 0.73725490196078436]  GraphicSpecularColor=[0.5 0.5 0.5 1.0]  GraphicAmbientColor=[0.15 0.15 0.15 1.0]  GraphicEmissiveColor=[0.0 0.0 0.0 1.0]  GraphicShininess=75  GraphicOpacity=1
  F : PMIOPort  Side=Left
  connections:
  Solid/RConn1 -- ReferenceFrame/RConn1 -- F/RConn1

== system multirotor_simulation/MULTIROTOR/3D/SIMECHANICS 3D SCENE/SimMechanics/MotorC/DCBL_Assembly_Clockwise_3_Top_1_RIGID/Assem3DCBL_Assembly_Clockwise_3_Top_1_RIGID/x10x4_7_clockwise_propeller_1_RIGID ==
  ReferenceFrame : sm_lib/Frames and Transforms/Reference Frame
  Solid : sm_lib/Body Elements/File Solid  ExtGeomFileName=10x4.7-clockwise-propeller_Default_sldprt.STL  UnitType=Custom  ExtGeomFileUnits=mm  StepReaderType=HEX  ExportConvexHullGeometry=off  InertiaType=Custom  Mass=0.0085886554018527825  MassUnits=kg  CenterOfMass=[5.0000101361481475 5.1432840109255382 3.799999228152465]  CenterOfMassUnits=mm  MomentsOfInertia=[37.986675876119939 39.040615812058284 1.1185316341050053]  MomentsOfInertiaUnits=kg*mm^2  ProductsOfInertia=[-7.8946012766185134e-07 -5.513228057178063 2.3221541821947674e-07]  ProductsOfInertiaUnits=kg*mm^2  BasedOnType=Density  Density=1000  DensityUnits=kg/(m^3)  DoExposeReferenceFrame=on  SerializedFrames=<Frames/>  GraphicType=FromGeometry  MarkerShape=Sphere  MarkerSize=10  MarkerSizeUnits=m  GraphicVisPropType=SimpleVisualProperties  GraphicDiffuseColor=[0.75294117647058822 0.75294117647058822 0.75294117647058822]  GraphicSpecularColor=[0.5 0.5 0.5 1.0]  GraphicAmbientColor=[0.15 0.15 0.15 1.0]  GraphicEmissiveColor=[0.0 0.0 0.0 1.0]  GraphicShininess=75  GraphicOpacity=1
  F : PMIOPort  Side=Left
  connections:
  Solid/RConn1 -- ReferenceFrame/RConn1 -- F/RConn1

== system multirotor_simulation/MULTIROTOR/3D/SIMECHANICS 3D SCENE/SimMechanics/MotorD/DCBL_Assembly_CounterClockwise_4_Top_1_RIGID/Assem4DCBL_Assembly_CounterClockwise_4_Top_1_RIGID/Mieng_chan_canh_quat_1_RIGID ==
  ReferenceFrame : sm_lib/Frames and Transforms/Reference Frame
  Solid : sm_lib/Body Elements/File Solid  ExtGeomFileName=Mieng_chan_canh_quat_Default_sldprt.STL  UnitType=Custom  ExtGeomFileUnits=mm  StepReaderType=HEX  ExportConvexHullGeometry=off  InertiaType=Custom  Mass=0.00066710164886432991  MassUnits=kg  CenterOfMass=[0 0.34100350204192958 0]  CenterOfMassUnits=mm  MomentsOfInertia=[0.0086037825507957657 0.016809111968954363 0.0086037825507957692]  MomentsOfInertiaUnits=kg*mm^2  ProductsOfInertia=[0 0 0]  ProductsOfInertiaUnits=kg*mm^2  BasedOnType=Density  Density=1000  DensityUnits=kg/(m^3)  DoExposeReferenceFrame=on  SerializedFrames=<Frames/>  GraphicType=FromGeometry  MarkerShape=Sphere  MarkerSize=10  MarkerSizeUnits=m  GraphicVisPropType=SimpleVisualProperties  GraphicDiffuseColor=[0.1 0.1 0.1]  GraphicSpecularColor=[0.5 0.5 0.5 1.0]  GraphicAmbientColor=[0.15 0.15 0.15 1.0]  GraphicEmissiveColor=[0.0 0.0 0.0 1.0]  GraphicShininess=75  GraphicOpacity=1
  F : PMIOPort  Side=Left
  connections:
  Solid/RConn1 -- ReferenceFrame/RConn1 -- F/RConn1

== system multirotor_simulation/MULTIROTOR/3D/SIMECHANICS 3D SCENE/SimMechanics/MotorD/DCBL_Assembly_CounterClockwise_4_Top_1_RIGID/Assem4DCBL_Assembly_CounterClockwise_4_Top_1_RIGID/Tang_tren_DCBL_1_RIGID ==
  ReferenceFrame : sm_lib/Frames and Transforms/Reference Frame
  Solid : sm_lib/Body Elements/File Solid  ExtGeomFileName=Tang_tren_DCBL_Default_sldprt.STL  UnitType=Custom  ExtGeomFileUnits=mm  StepReaderType=HEX  ExportConvexHullGeometry=off  InertiaType=Custom  Mass=0.0096533797201190392  MassUnits=kg  CenterOfMass=[0 -3.2502099324489322 0]  CenterOfMassUnits=mm  MomentsOfInertia=[1.2743807926810715 0.81038583319969226 1.2743807926810709]  MomentsOfInertiaUnits=kg*mm^2  ProductsOfInertia=[0 0 0]  ProductsOfInertiaUnits=kg*mm^2  BasedOnType=Density  Density=1000  DensityUnits=kg/(m^3)  DoExposeReferenceFrame=on  SerializedFrames=<Frames/>  GraphicType=FromGeometry  MarkerShape=Sphere  MarkerSize=10  MarkerSizeUnits=m  GraphicVisPropType=SimpleVisualProperties  GraphicDiffuseColor=[0.1 0.1 0.1]  GraphicSpecularColor=[0.5 0.5 0.5 1.0]  GraphicAmbientColor=[0.15 0.15 0.15 1.0]  GraphicEmissiveColor=[0.0 0.0 0.0 1.0]  GraphicShininess=75  GraphicOpacity=1
  F : PMIOPort  Side=Left
  connections:
  Solid/RConn1 -- ReferenceFrame/RConn1 -- F/RConn1

== system multirotor_simulation/MULTIROTOR/3D/SIMECHANICS 3D SCENE/SimMechanics/MotorD/DCBL_Assembly_CounterClockwise_4_Top_1_RIGID/Assem4DCBL_Assembly_CounterClockwise_4_Top_1_RIGID/hex_nut_style_1_gradeab_iso_1_RIGID ==
  ReferenceFrame : sm_lib/Frames and Transforms/Reference Frame
  Solid : sm_lib/Body Elements/File Solid  ExtGeomFileName=hex nut style 1 gradeab_iso_Hexagon Nut ISO - 4032 - M4 - D - N_sldprt.STL  UnitType=Custom  ExtGeomFileUnits=mm  StepReaderType=HEX  ExportConvexHullGeometry=off  InertiaType=Custom  Mass=0.00010662444846940384  MassUnits=kg  CenterOfMass=[0 1.3702747535691162e-06 -1.5985959803450969]  CenterOfMassUnits=mm  MomentsOfInertia=[0.00052487586358693401 0.00052487294180577238 0.00087302244809774987]  MomentsOfInertiaUnits=kg*mm^2  ProductsOfInertia=[0 0 0]  ProductsOfInertiaUnits=kg*mm^2  BasedOnType=Density  Density=1000  DensityUnits=kg/(m^3)  DoExposeReferenceFrame=on  SerializedFrames=<Frames/>  GraphicType=FromGeometry  MarkerShape=Sphere  MarkerSize=10  MarkerSizeUnits=m  GraphicVisPropType=SimpleVisualProperties  GraphicDiffuseColor=[0.77647058823529413 0.75686274509803919 0.73725490196078436]  GraphicSpecularColor=[0.5 0.5 0.5 1.0]  GraphicAmbientColor=[0.15 0.15 0.15 1.0]  GraphicEmissiveColor=[0.0 0.0 0.0 1.0]  GraphicShininess=75  GraphicOpacity=1
  F : PMIOPort  Side=Left
  connections:
  Solid/RConn1 -- ReferenceFrame/RConn1 -- F/RConn1

== system multirotor_simulation/MULTIROTOR/3D/SIMECHANICS 3D SCENE/SimMechanics/MotorD/DCBL_Assembly_CounterClockwise_4_Top_1_RIGID/Assem4DCBL_Assembly_CounterClockwise_4_Top_1_RIGID/x10x4_7_counterclockwise_propeller_1_RIGID ==
  ReferenceFrame : sm_lib/Frames and Transforms/Reference Frame
  Solid : sm_lib/Body Elements/File Solid  ExtGeomFileName=10x4.7-counterclockwise-propeller_Default_sldprt.STL  UnitType=Custom  ExtGeomFileUnits=mm  StepReaderType=HEX  ExportConvexHullGeometry=off  InertiaType=Custom  Mass=0.0086221636611543556  MassUnits=kg  CenterOfMass=[5.0000063702530122 5.136767030722547 3.7999863031218535]  CenterOfMassUnits=mm  MomentsOfInertia=[38.086408780943664 39.145966882895458 1.124519086575168]  MomentsOfInertiaUnits=kg*mm^2  ProductsOfInertia=[-1.7703894482553841e-07 5.5344154529569156 1.457353668708178e-07]  ProductsOfInertiaUnits=kg*mm^2  BasedOnType=Density  Density=1000  DensityUnits=kg/(m^3)  DoExposeReferenceFrame=on  SerializedFrames=<Frames/>  GraphicType=FromGeometry  MarkerShape=Sphere  MarkerSize=10  MarkerSizeUnits=m  GraphicVisPropType=SimpleVisualProperties  GraphicDiffuseColor=[0.75294117647058822 0.75294117647058822 0.75294117647058822]  GraphicSpecularColor=[0.5 0.5 0.5 1.0]  GraphicAmbientColor=[0.15 0.15 0.15 1.0]  GraphicEmissiveColor=[0.0 0.0 0.0 1.0]  GraphicShininess=75  GraphicOpacity=1
  F : PMIOPort  Side=Left
  connections:
  Solid/RConn1 -- ReferenceFrame/RConn1 -- F/RConn1

== matlab function multirotor_simulation/MULTIROTOR/MULTIPLE ROTORS FORCES AND MOMENTS/Subsystem1/MATLAB Function ==
  data: Q input; Pe output; Omega input; p00 input; p10 input; p01 input; p20 input; p11 input; p02 input
function Pe  = fcn(Q, Omega, p00, p10, p01, p20, p11, p02)
eta_e = p00 + p10*Omega  +p01*Q + p20*Omega^2 + p11*Omega*Q + p02*Q^2;
Psh = Omega*Q;
Pe=Psh/eta_e;

== matlab function multirotor_simulation/MULTIROTOR/MULTIPLE ROTORS FORCES AND MOMENTS/Subsystem1/NASA TM84281 ==
  data: BLADES input; F_rotor output; ASLOPE input; CHORD input; CHORD75 input; ROTOR input; a0 input; Theta0 input; THETT input; dyn_visco input; k_ind input; STACG input; BLCG input; WLCG input; STAH input; BLH input; WLH input; chi input; rho input; TAS input; omega_TAS input; Omega input; M_rotor output; Q output; vi output; lambda output; omega input; g input; h input
function [F_rotor, M_rotor, Q, vi, lambda] = fcn(BLADES, ASLOPE, CHORD, CHORD75, ROTOR, a0, Theta0, THETT, dyn_visco, k_ind, STACG, BLCG, WLCG, STAH, BLH, WLH, chi, rho, TAS, omega_TAS, Omega, omega, g, h)

%% Preliminary calculations
A = pi*ROTOR^2;
sigma = BLADES*CHORD/(pi*ROTOR);
lever_arm_H = [STACG-STAH BLH-BLCG WLCG-WLH]'; %STA-line and W-line against coordinate sys
TAS_H = [1 chi 1]'.*(TAS + cross(omega_TAS, lever_arm_H));
uH = TAS_H(1);
vH = TAS_H(2);
wH = TAS_H(3);
betta_w = atan2(vH, uH);
Mu = sqrt(uH^2+vH^2)/(Omega*ROTOR); %Ratio between the in -plane speed and the tip speed
p = omega(1); %Body Frame Roll-Rate
q = omega(2); %Body Frame Pitch-Ratw
pH = chi*p; %Hub Frame
qH = q; %Hub Frame
%Omega: scalar rate of rotor
%omega: rotation rate of MR

%% thrust calculations
lambda = fzero(@(x) x-wH/(Omega*ROTOR) + 0.5*((0.5*BLADES*rho*ASLOPE*CHORD*ROTOR*(Omega*ROTOR)^2*(x/2 + Theta0*(1/3+Mu^2/2) + THETT*(1/4+Mu^2/4) + Mu/4*(pH/Omega*cos(betta_w)+qH/Omega*sin(betta_w))))/(rho*A*(Omega*ROTOR)^2))/sqrt(Mu^2+x^2), -0.1);
T = (0.5*BLADES*rho*ASLOPE*CHORD*ROTOR*(Omega*ROTOR)^2*(lambda/2 + Theta0*(1/3+Mu^2/2) + THETT*(1/4+Mu^2/4) + Mu/4*(pH/Omega*cos(betta_w)+qH/Omega*sin(betta_w))));

%T = @(x)(0.5*BLADES*rho*ASLOPE*CHORD*ROTOR*(Omega*ROTOR)^2*(x/2 + Theta0*(1/3+Mu^2/2) + THETT*(1/4+Mu^2/4) + Mu/4*(pH/Omega*cos(betta_w)+qH/Omega*sin(betta_w))));
%lambda = fzero(@(x) x-wH/(Omega*ROTOR) + 0.5*(T(x)/(rho*A*(Omega*ROTOR)^2))/sqrt(Mu^2+x^2), -0.1);
%T = T(lambda);

vi = wH-lambda*Omega*ROTOR;

CT = T/(rho*A*(Omega*ROTOR)^2);
V75 = sqrt(vi^2+(0.75*Omega*ROTOR)^2);
Re = (rho*CHORD75*V75)/dyn_visco;
delta = 0.1166*Re^(-0.2) + 0.3/ASLOPE^2*(6*CT/sigma/(1+3/2*Mu^2))^2;

%% other forces and moments in the hub-wind frame
H_w=0.5*BLADES*rho*ASLOPE*CHORD*ROTOR*(Omega*ROTOR)^2 *((delta*Mu/(2*ASLOPE))-Theta0/4*(2*lambda*Mu +2/3*(pH/Omega *cos(betta_w) + qH/Omega *sin(betta_w))) - THETT/4*( Mu*lambda +0.5*(pH/Omega *cos(betta_w) + qH/Omega *sin(betta_w))) -0.25*(2/3*a0*(-pH/Omega *sin(betta_w)+ qH/Omega *cos(betta_w)) -2*lambda*(pH/Omega *cos(betta_w) + qH/Omega *sin(betta_w))) +0.25*Mu*a0^2);
Y_w=0.5*BLADES*rho*ASLOPE*CHORD*ROTOR*(Omega*ROTOR)^2 * (-0.25*Theta0*(3*a0*Mu- 2/3*(-pH/Omega *sin(betta_w)+qH/Omega *cos(betta_w))) -0.25*THETT*(2*a0*Mu -0.5*(-pH/Omega *sin(betta_w)+qH/Omega *cos(betta_w))) -0.25*6*Mu*a0*lambda);
L_w = 0;
M_w = 0;
Q=k_ind*(0.5*BLADES*rho*ASLOPE*CHORD*ROTOR^2*(Omega*ROTOR)^2*(delta/(4*ASLOPE*k_ind) *(1+Mu^2) -Theta0*(lambda/3 + Mu/6 *(pH/Omega *cos(betta_w) + qH/Omega *sin(betta_w))) -THETT*lambda*0.25 -0.5*(lambda^2 + Mu^2*(0.5*a0^2)) +Mu*a0/3*(-pH/Omega*sin(betta_w) +qH/Omega *cos(betta_w)) -1/8*(-pH/Omega*sin(betta_w) +qH/Omega *cos(betta_w))^2 -1/8*(pH/Omega *cos(betta_w) + qH/Omega *sin(betta_w))));

%% back rotation from hub-wind frame to hub frame
H_H = H_w*cos(betta_w) + Y_w*sin(betta_w);
Y_H = -H_w*sin(betta_w) + Y_w*cos(betta_w);
L_H = L_w*cos(betta_w) - M_w*sin(betta_w);
M_H = L_w*sin(betta_w) + M_w*cos(betta_w);

%% back rotation from hub frame to body frame
X = -H_H;
Y = chi*Y_H;
Z = -T;
F_rotor = [X Y Z]';
M_rotor = [chi*L_H M_H chi*Q]' + cross(lever_arm_H, F_rotor);

== matlab function multirotor_simulation/MULTIROTOR/MULTIPLE ROTORS FORCES AND MOMENTS/Subsystem2/MATLAB Function ==
  data: Q input; Pe output; Omega input; p00 input; p10 input; p01 input; p20 input; p11 input; p02 input
function Pe  = fcn(Q, Omega, p00, p10, p01, p20, p11, p02)
eta_e = p00 + p10*Omega  +p01*Q + p20*Omega^2 + p11*Omega*Q + p02*Q^2;
Psh = Omega*Q;
Pe=Psh/eta_e;

== matlab function multirotor_simulation/MULTIROTOR/MULTIPLE ROTORS FORCES AND MOMENTS/Subsystem2/NASA TM84281 ==
  data: BLADES input; F_rotor output; ASLOPE input; CHORD input; CHORD75 input; ROTOR input; a0 input; Theta0 input; THETT input; dyn_visco input; k_ind input; STACG input; BLCG input; WLCG input; STAH input; BLH input; WLH input; chi input; rho input; TAS input; omega_TAS input; Omega input; M_rotor output; Q output; vi output; lambda output; omega input; g input; h input
function [F_rotor, M_rotor, Q, vi, lambda] = fcn(BLADES, ASLOPE, CHORD, CHORD75, ROTOR, a0, Theta0, THETT, dyn_visco, k_ind, STACG, BLCG, WLCG, STAH, BLH, WLH, chi, rho, TAS, omega_TAS, Omega, omega, g, h)

%% Preliminary calculations
A = pi*ROTOR^2;
sigma = BLADES*CHORD/(pi*ROTOR);
lever_arm_H = [STACG-STAH BLH-BLCG WLCG-WLH]'; %STA-line and W-line against coordinate sys
TAS_H = [1 chi 1]'.*(TAS + cross(omega_TAS, lever_arm_H));
uH = TAS_H(1);
vH = TAS_H(2);
wH = TAS_H(3);
betta_w = atan2(vH, uH);
Mu = sqrt(uH^2+vH^2)/(Omega*ROTOR); %Ratio between the in -plane speed and the tip speed
p = omega(1); %Body Frame Roll-Rate
q = omega(2); %Body Frame Pitch-Ratw
pH = chi*p; %Hub Frame
qH = q; %Hub Frame
%Omega: scalar rate of rotor
%omega: rotation rate of MR

%% thrust calculations
lambda = fzero(@(x) x-wH/(Omega*ROTOR) + 0.5*((0.5*BLADES*rho*ASLOPE*CHORD*ROTOR*(Omega*ROTOR)^2*(x/2 + Theta0*(1/3+Mu^2/2) + THETT*(1/4+Mu^2/4) + Mu/4*(pH/Omega*cos(betta_w)+qH/Omega*sin(betta_w))))/(rho*A*(Omega*ROTOR)^2))/sqrt(Mu^2+x^2), -0.1);
T = (0.5*BLADES*rho*ASLOPE*CHORD*ROTOR*(Omega*ROTOR)^2*(lambda/2 + Theta0*(1/3+Mu^2/2) + THETT*(1/4+Mu^2/4) + Mu/4*(pH/Omega*cos(betta_w)+qH/Omega*sin(betta_w))));

%T = @(x)(0.5*BLADES*rho*ASLOPE*CHORD*ROTOR*(Omega*ROTOR)^2*(x/2 + Theta0*(1/3+Mu^2/2) + THETT*(1/4+Mu^2/4) + Mu/4*(pH/Omega*cos(betta_w)+qH/Omega*sin(betta_w))));
%lambda = fzero(@(x) x-wH/(Omega*ROTOR) + 0.5*(T(x)/(rho*A*(Omega*ROTOR)^2))/sqrt(Mu^2+x^2), -0.1);
%T = T(lambda);

vi = wH-lambda*Omega*ROTOR;

CT = T/(rho*A*(Omega*ROTOR)^2);
V75 = sqrt(vi^2+(0.75*Omega*ROTOR)^2);
Re = (rho*CHORD75*V75)/dyn_visco;
delta = 0.1166*Re^(-0.2) + 0.3/ASLOPE^2*(6*CT/sigma/(1+3/2*Mu^2))^2;

%% other forces and moments in the hub-wind frame
H_w=0.5*BLADES*rho*ASLOPE*CHORD*ROTOR*(Omega*ROTOR)^2 *((delta*Mu/(2*ASLOPE))-Theta0/4*(2*lambda*Mu +2/3*(pH/Omega *cos(betta_w) + qH/Omega *sin(betta_w))) - THETT/4*( Mu*lambda +0.5*(pH/Omega *cos(betta_w) + qH/Omega *sin(betta_w))) -0.25*(2/3*a0*(-pH/Omega *sin(betta_w)+ qH/Omega *cos(betta_w)) -2*lambda*(pH/Omega *cos(betta_w) + qH/Omega *sin(betta_w))) +0.25*Mu*a0^2);
Y_w=0.5*BLADES*rho*ASLOPE*CHORD*ROTOR*(Omega*ROTOR)^2 * (-0.25*Theta0*(3*a0*Mu- 2/3*(-pH/Omega *sin(betta_w)+qH/Omega *cos(betta_w))) -0.25*THETT*(2*a0*Mu -0.5*(-pH/Omega *sin(betta_w)+qH/Omega *cos(betta_w))) -0.25*6*Mu*a0*lambda);
L_w = 0;
M_w = 0;
Q=k_ind*(0.5*BLADES*rho*ASLOPE*CHORD*ROTOR^2*(Omega*ROTOR)^2*(delta/(4*ASLOPE*k_ind) *(1+Mu^2) -Theta0*(lambda/3 + Mu/6 *(pH/Omega *cos(betta_w) + qH/Omega *sin(betta_w))) -THETT*lambda*0.25 -0.5*(lambda^2 + Mu^2*(0.5*a0^2)) +Mu*a0/3*(-pH/Omega*sin(betta_w) +qH/Omega *cos(betta_w)) -1/8*(-pH/Omega*sin(betta_w) +qH/Omega *cos(betta_w))^2 -1/8*(pH/Omega *cos(betta_w) + qH/Omega *sin(betta_w))));

%% back rotation from hub-wind frame to hub frame
H_H = H_w*cos(betta_w) + Y_w*sin(betta_w);
Y_H = -H_w*sin(betta_w) + Y_w*cos(betta_w);
L_H = L_w*cos(betta_w) - M_w*sin(betta_w);
M_H = L_w*sin(betta_w) + M_w*cos(betta_w);

%% back rotation from hub frame to body frame
X = -H_H;
Y = chi*Y_H;
Z = -T;
F_rotor = [X Y Z]';
M_rotor = [chi*L_H M_H chi*Q]' + cross(lever_arm_H, F_rotor);
